simulink model "CC_CV_IR"  (R2019b)
settings: Solver=ode23s  StartTime=0.0  StopTime=96  FixedStep=50e-6  RelTol=1e-6
libraries: powerlib x14, simulink x6
settings Model: Creator=Soto Porras  LastModifiedBy=maxim
settings DataIOCC: ReturnWorkspaceOutputs=off
settings DebuggingCC: ArithmeticOperatorsInVariantConditions=warning
settings SFSimCC: CustomCodeUndefinedFunction=UseInterfaceOnly

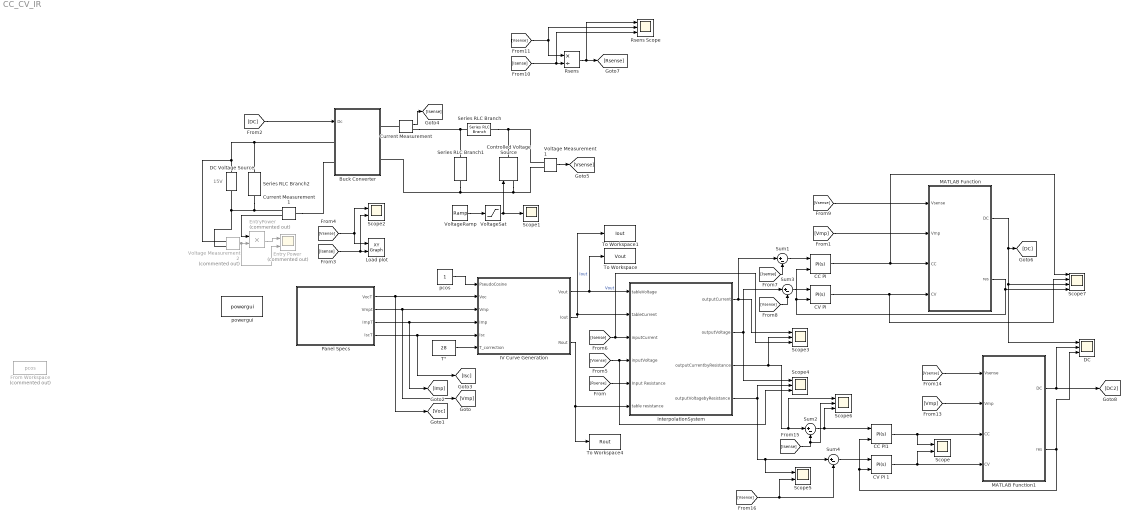
== system CC_CV_IR ==
  note: 15V
  Buck Converter : Subsystem
  CC PI : simulink/Continuous/PID Controller  Controller=PI  Form=Parallel  TimeDomain=Continuous-time  SampleTime=0.00005  IntegratorMethod=Trapezoidal  FilterMethod=Forward Euler  ControllerParametersSource=internal  P=10  I=0.01  D=0  UseFilter=on  N=100  TunerSelectOption=Frequency Response Based  InitialConditionSource=internal  InitialConditionForIntegrator=0  InitialConditionForFilter=0  DifferentiatorICPrevScaledInput=0  ExternalReset=either  TrackingMode=off  Kt=1  LimitOutput=off  UpperSaturationLimit=0.9  LowerSaturationLimit=0.1  LinearizeAsGain=on  AntiWindupMode=none  Kb=1  POutMin=[]  POutMax=[]  IOutMin=[]  IOutMax=[]  DOutMin=[]  DOutMax=[]  NOutMin=[]  NOutMax=[]  SumOutMin=[]  SumOutMax=[]  SaturationOutMin=[]  SaturationOutMax=[]  PParamMin=[]  PParamMax=[]  IParamMin=[]  IParamMax=[]  DParamMin=[]  DParamMax=[]  NParamMin=[]  NParamMax=[]  KbParamMin=[]  KbParamMax=[]  KtParamMin=[]  KtParamMax=[]  KbOutMin=[]  KbOutMax=[]  KtOutMin=[]  KtOutMax=[]  IntegratorOutMin=[]  IntegratorOutMax=[]  FilterOutMin=[]  FilterOutMax=[]  SumI1OutMin=[]  SumI1OutMax=[]  SumI2OutMin=[]  SumI2OutMax=[]  SumI3OutMin=[]  SumI3OutMax=[]  SumI4OutMin=[]  SumI4OutMax=[]  SumDOutMin=[]  SumDOutMax=[]  DifferentiatorOutMin=[]  DifferentiatorOutMax=[]  FilterDiffOutCoefMin=[]  FilterDiffOutCoefMax=[]  ReciprocalOutMin=[]  ReciprocalOutMax=[]  SumDenOutMin=[]  SumDenOutMax=[]  SumNumOutMin=[]  SumNumOutMax=[]  DivideOutMin=[]  DivideOutMax=[]  IntegratorContinuousStateAttributes=''  IntegratorStateMustResolveToSignalObject=off  IntegratorRTWStateStorageClass=Auto  FilterContinuousStateAttributes=''  FilterStateMustResolveToSignalObject=off  FilterRTWStateStorageClass=Auto  ParallelPVariant=InternalParameters  IdealPVariant=Disabled  IVariant=InternalParameters  DVariant=Disabled  IntegratorVariant=Continuous  SatVariant=Disabled  AWVariant=Passthrough  PCopyVariant=Disabled  TRVariant=Disabled  FdbkBlocksVariant=Forward  IdealPFdbkVariant=Disabled  SatFdbkVariant=Disabled  DerivativeFilterVariant=Disabled  NVariant=Disabled  NCopyVariant=Disabled_SignalSpec  FilterICVariant=Disabled  IntegratorICVariant=InternalICs  ExternalResetVariant=ExternalReset  TRSumVariant=Passthrough  SumFdbkVariant=Disabled  SumVariant=Sum_PI
  CC PI1 : simulink/Continuous/PID Controller  Controller=PI  Form=Parallel  TimeDomain=Continuous-time  SampleTime=0.00005  IntegratorMethod=Trapezoidal  FilterMethod=Forward Euler  ControllerParametersSource=internal  P=5  I=0.0001  D=0  UseFilter=on  N=100  TunerSelectOption=Frequency Response Based  InitialConditionSource=internal  InitialConditionForIntegrator=0  InitialConditionForFilter=0  DifferentiatorICPrevScaledInput=0  ExternalReset=either  TrackingMode=off  Kt=1  LimitOutput=off  UpperSaturationLimit=0.9  LowerSaturationLimit=0.1  LinearizeAsGain=on  AntiWindupMode=none  Kb=1  POutMin=[]  POutMax=[]  IOutMin=[]  IOutMax=[]  DOutMin=[]  DOutMax=[]  NOutMin=[]  NOutMax=[]  SumOutMin=[]  SumOutMax=[]  SaturationOutMin=[]  SaturationOutMax=[]  PParamMin=[]  PParamMax=[]  IParamMin=[]  IParamMax=[]  DParamMin=[]  DParamMax=[]  NParamMin=[]  NParamMax=[]  KbParamMin=[]  KbParamMax=[]  KtParamMin=[]  KtParamMax=[]  KbOutMin=[]  KbOutMax=[]  KtOutMin=[]  KtOutMax=[]  IntegratorOutMin=[]  IntegratorOutMax=[]  FilterOutMin=[]  FilterOutMax=[]  SumI1OutMin=[]  SumI1OutMax=[]  SumI2OutMin=[]  SumI2OutMax=[]  SumI3OutMin=[]  SumI3OutMax=[]  SumI4OutMin=[]  SumI4OutMax=[]  SumDOutMin=[]  SumDOutMax=[]  DifferentiatorOutMin=[]  DifferentiatorOutMax=[]  FilterDiffOutCoefMin=[]  FilterDiffOutCoefMax=[]  ReciprocalOutMin=[]  ReciprocalOutMax=[]  SumDenOutMin=[]  SumDenOutMax=[]  SumNumOutMin=[]  SumNumOutMax=[]  DivideOutMin=[]  DivideOutMax=[]  IntegratorContinuousStateAttributes=''  IntegratorStateMustResolveToSignalObject=off  IntegratorRTWStateStorageClass=Auto  FilterContinuousStateAttributes=''  FilterStateMustResolveToSignalObject=off  FilterRTWStateStorageClass=Auto  ParallelPVariant=InternalParameters  IdealPVariant=Disabled  IVariant=InternalParameters  DVariant=Disabled  IntegratorVariant=Continuous  SatVariant=Disabled  AWVariant=Passthrough  PCopyVariant=Disabled  TRVariant=Disabled  FdbkBlocksVariant=Forward  IdealPFdbkVariant=Disabled  SatFdbkVariant=Disabled  DerivativeFilterVariant=Disabled  NVariant=Disabled  NCopyVariant=Disabled_SignalSpec  FilterICVariant=Disabled  IntegratorICVariant=InternalICs  ExternalResetVariant=ExternalReset  TRSumVariant=Passthrough  SumFdbkVariant=Disabled  SumVariant=Sum_PI
  "CV PI " : simulink/Continuous/PID Controller  Controller=PI  Form=Parallel  TimeDomain=Continuous-time  SampleTime=0.00005  IntegratorMethod=Trapezoidal  FilterMethod=Forward Euler  ControllerParametersSource=internal  P=10  I=0.1  D=0.01  UseFilter=on  N=100  TunerSelectOption=Transfer Function Based (PID Tuner App)  InitialConditionSource=internal  InitialConditionForIntegrator=0  InitialConditionForFilter=0  DifferentiatorICPrevScaledInput=0  ExternalReset=either  TrackingMode=off  Kt=1  LimitOutput=off  UpperSaturationLimit=0.9  LowerSaturationLimit=0.1  LinearizeAsGain=on  AntiWindupMode=none  Kb=1  POutMin=[]  POutMax=[]  IOutMin=[]  IOutMax=[]  DOutMin=[]  DOutMax=[]  NOutMin=[]  NOutMax=[]  SumOutMin=[]  SumOutMax=[]  SaturationOutMin=[]  SaturationOutMax=[]  PParamMin=[]  PParamMax=[]  IParamMin=[]  IParamMax=[]  DParamMin=[]  DParamMax=[]  NParamMin=[]  NParamMax=[]  KbParamMin=[]  KbParamMax=[]  KtParamMin=[]  KtParamMax=[]  KbOutMin=[]  KbOutMax=[]  KtOutMin=[]  KtOutMax=[]  IntegratorOutMin=[]  IntegratorOutMax=[]  FilterOutMin=[]  FilterOutMax=[]  SumI1OutMin=[]  SumI1OutMax=[]  SumI2OutMin=[]  SumI2OutMax=[]  SumI3OutMin=[]  SumI3OutMax=[]  SumI4OutMin=[]  SumI4OutMax=[]  SumDOutMin=[]  SumDOutMax=[]  DifferentiatorOutMin=[]  DifferentiatorOutMax=[]  FilterDiffOutCoefMin=[]  FilterDiffOutCoefMax=[]  ReciprocalOutMin=[]  ReciprocalOutMax=[]  SumDenOutMin=[]  SumDenOutMax=[]  SumNumOutMin=[]  SumNumOutMax=[]  DivideOutMin=[]  DivideOutMax=[]  IntegratorContinuousStateAttributes=''  IntegratorStateMustResolveToSignalObject=off  IntegratorRTWStateStorageClass=Auto  FilterContinuousStateAttributes=''  FilterStateMustResolveToSignalObject=off  FilterRTWStateStorageClass=Auto  ParallelPVariant=InternalParameters  IdealPVariant=Disabled  IVariant=InternalParameters  DVariant=Disabled  IntegratorVariant=Continuous  SatVariant=Disabled  AWVariant=Passthrough  PCopyVariant=Disabled  TRVariant=Disabled  FdbkBlocksVariant=Forward  IdealPFdbkVariant=Disabled  SatFdbkVariant=Disabled  DerivativeFilterVariant=Disabled  NVariant=Disabled  NCopyVariant=Disabled_SignalSpec  FilterICVariant=Disabled  IntegratorICVariant=InternalICs  ExternalResetVariant=ExternalReset  TRSumVariant=Passthrough  SumFdbkVariant=Disabled  SumVariant=Sum_PI
  CV PI 1 : simulink/Continuous/PID Controller  Controller=PI  Form=Parallel  TimeDomain=Continuous-time  SampleTime=0.00005  IntegratorMethod=Trapezoidal  FilterMethod=Forward Euler  ControllerParametersSource=internal  P=10  I=0.0001  D=0.01  UseFilter=on  N=100  TunerSelectOption=Transfer Function Based (PID Tuner App)  InitialConditionSource=internal  InitialConditionForIntegrator=0  InitialConditionForFilter=0  DifferentiatorICPrevScaledInput=0  ExternalReset=either  TrackingMode=off  Kt=1  LimitOutput=off  UpperSaturationLimit=0.9  LowerSaturationLimit=0.1  LinearizeAsGain=on  AntiWindupMode=none  Kb=1  POutMin=[]  POutMax=[]  IOutMin=[]  IOutMax=[]  DOutMin=[]  DOutMax=[]  NOutMin=[]  NOutMax=[]  SumOutMin=[]  SumOutMax=[]  SaturationOutMin=[]  SaturationOutMax=[]  PParamMin=[]  PParamMax=[]  IParamMin=[]  IParamMax=[]  DParamMin=[]  DParamMax=[]  NParamMin=[]  NParamMax=[]  KbParamMin=[]  KbParamMax=[]  KtParamMin=[]  KtParamMax=[]  KbOutMin=[]  KbOutMax=[]  KtOutMin=[]  KtOutMax=[]  IntegratorOutMin=[]  IntegratorOutMax=[]  FilterOutMin=[]  FilterOutMax=[]  SumI1OutMin=[]  SumI1OutMax=[]  SumI2OutMin=[]  SumI2OutMax=[]  SumI3OutMin=[]  SumI3OutMax=[]  SumI4OutMin=[]  SumI4OutMax=[]  SumDOutMin=[]  SumDOutMax=[]  DifferentiatorOutMin=[]  DifferentiatorOutMax=[]  FilterDiffOutCoefMin=[]  FilterDiffOutCoefMax=[]  ReciprocalOutMin=[]  ReciprocalOutMax=[]  SumDenOutMin=[]  SumDenOutMax=[]  SumNumOutMin=[]  SumNumOutMax=[]  DivideOutMin=[]  DivideOutMax=[]  IntegratorContinuousStateAttributes=''  IntegratorStateMustResolveToSignalObject=off  IntegratorRTWStateStorageClass=Auto  FilterContinuousStateAttributes=''  FilterStateMustResolveToSignalObject=off  FilterRTWStateStorageClass=Auto  ParallelPVariant=InternalParameters  IdealPVariant=Disabled  IVariant=InternalParameters  DVariant=Disabled  IntegratorVariant=Continuous  SatVariant=Disabled  AWVariant=Passthrough  PCopyVariant=Disabled  TRVariant=Disabled  FdbkBlocksVariant=Forward  IdealPFdbkVariant=Disabled  SatFdbkVariant=Disabled  DerivativeFilterVariant=Disabled  NVariant=Disabled  NCopyVariant=Disabled_SignalSpec  FilterICVariant=Disabled  IntegratorICVariant=InternalICs  ExternalResetVariant=ExternalReset  TRSumVariant=Passthrough  SumFdbkVariant=Disabled  SumVariant=Sum_PI
  Controlled Voltage Source : powerlib/Electrical Sources/Controlled Voltage Source  Initialize=on  Source_Type=DC  Amplitude=0.1  Phase=0  Frequency=0  Measurements=None
      settings: SourceProductName=Simscape Electrical
  Current Measurement : powerlib/Measurements/Current Measurement  PhasorSimulation=off  OutputType=Complex  PSBequivalent=0
      settings: SourceProductName=Simscape Electrical
  Current Measurement1 : powerlib/Measurements/Current Measurement  PhasorSimulation=off  OutputType=Complex  PSBequivalent=0
      settings: SourceProductName=Simscape Electrical
  "DC " : Scope  NumInputPorts=3
  DC Voltage Source : powerlib/Electrical Sources/DC Voltage Source  Amplitude=15  Measurements=None
      settings: SourceProductName=Simscape Electrical
  "Entry Power " : Scope  Commented=on  NumInputPorts=2
  EntryPower : Product  Commented=on
  From Workspace : FromWorkspace  Commented=on  VariableName=pcos  SampleTime=0
  IV Curve Generation : Subsystem  mask(Panel I-V Curve Calculation){ValueVocComp=0.0062, ValueVmpComp=0.0067}
      mask prompts: ValueVocComp "Voc Temperature Correction (V)"; ValueVmpComp "Vmp Temperature Correction (V)"
      mask help:
      | This module calculates the panel IV curve using the next panel parameters:
      | 1. Voc
      | 2. Vmp
      | 3. Imp
      | 4. Isc
      |
      | It applies:
      | 1. Correction to current parameters (Isc and Imp) using a pseudo cosine that varies depending on the angle of the perpendicular CubeSat face and the sun's incident radiation.
      | 2. Correction to voltage parameters (Voc and Vmp) using the panel datasheet voltage losses, given in V by the user.
      mask TypeOptions ValueVocComp: Voc_comp/Value
      mask TypeOptions ValueVmpComp: Vmp_comp/Value
      mask Display: image('IV_curve.png');
  InterpolationSystem : Subsystem
  Load plot : simulink/Sinks/XY Graph  xmin=0  xmax=6  ymin=0  ymax=2  st=-1
  MATLAB Function : MATLAB Function  TreatAsAtomicUnit=on
  MATLAB Function1 : MATLAB Function  TreatAsAtomicUnit=on
  Panel Specs : Subsystem  mask(Solar Panel Specifications){Voc=2.690, Vmp=2.409, Imp=0.5029, Isc=0.5196, SerialGain=2, ParallelGain=3}
      mask prompts: SerialGain "Serial"; ParallelGain "Parallel"
      mask help: Inputs solar panel electrical specifications, temperature and array distribution.
      mask TypeOptions Voc: Voc/Value
      mask TypeOptions Vmp: Vmp/Value
      mask TypeOptions Imp: Imp/Value
      mask TypeOptions Isc: Isc/Value
      mask TypeOptions SerialGain: Gain/Gain | Gain1/Gain
      mask TypeOptions ParallelGain: Gain2/Gain | Gain3/Gain
      mask DialogControl Container3 Prompt: Panel Array
      mask Display: image('solar_panel.png');
  Rsens : Product  Inputs=*/
  Rsens Scope : Scope  NumInputPorts=3
  Scope : Scope  NumInputPorts=2
  Scope1 : Scope
  Scope2 : Scope  NumInputPorts=2
  Scope3 : Scope  NumInputPorts=3
  Scope4 : Scope  NumInputPorts=3
  Scope5 : Scope  NumInputPorts=2
  Scope6 : Scope  NumInputPorts=3
  Scope7 : Scope  NumInputPorts=4
  Series RLC Branch : powerlib/Elements/Series RLC Branch  LConnTagsString=__new0  RConnTagsString=__new0  BranchType=R  Resistance=1e-3  Inductance=1e-3  SetiL0=off  InitialCurrent=0  Capacitance=1e-6  Setx0=off  InitialVoltage=0  Measurements=None
      settings: SourceProductName=Simscape Electrical
  Series RLC Branch1 : powerlib/Elements/Series RLC Branch  LConnTagsString=__new0  RConnTagsString=__new0  BranchType=RC  Resistance=1e-2  Inductance=1e-3  SetiL0=off  InitialCurrent=0  Capacitance=100e-6  Setx0=off  InitialVoltage=0  Measurements=None
      settings: SourceProductName=Simscape Electrical
  Series RLC Branch2 : powerlib/Elements/Series RLC Branch  LConnTagsString=__new0  RConnTagsString=__new0  BranchType=RC  Resistance=1e-3  Inductance=1e-3  SetiL0=off  InitialCurrent=0  Capacitance=100e-6  Setx0=off  InitialVoltage=0  Measurements=None
      settings: SourceProductName=Simscape Electrical
  Sum{1..4} (4 alike) : Sum  Inputs=|+-
  To Workspace : ToWorkspace  VariableName=Vout  SaveFormat=Structure With Time  SampleTime=-1
  To Workspace1 : ToWorkspace  VariableName=Iout  SaveFormat=Structure With Time  SampleTime=-1
  To Workspace4 : ToWorkspace  VariableName=Rout  SaveFormat=Structure With Time  SampleTime=-1
  T° : Constant  Value=28
  Voltage Measurement1 : powerlib/Measurements/Voltage Measurement  PhasorSimulation=off  OutputType=Complex  PSBequivalent=0
      settings: SourceProductName=Simscape Electrical
  Voltage Measurement2 : powerlib/Measurements/Voltage Measurement  Commented=on  PhasorSimulation=off  OutputType=Complex  PSBequivalent=0
      settings: SourceProductName=Simscape Electrical
  VoltageRamp : simulink/Sources/Ramp  slope=0.0538  start=0  InitialOutput=0
  VoltageSat : Saturate  UpperLimit=5.38  LowerLimit=0
  pcos : Constant
  powergui : powerlib/powergui  Priority=1  SimulationMode=Continuous  SampleTime=50e-6  frequency=60  Iterations=50  frequencyindice=0  Pbase=100e6  ErrMax=1e-4  UnitsV=kV  UnitsW=MW  buscounter=0  FunctionMessages=off  echomessages=off  EnableUseOfTLC=off  CurrentSourceSwitches=off  DisableSnubberDevices=off  DisableRonSwitches=off  DisableVfSwitches=off  DisplayEquations=off  AutomaticDiscreteSolvers=off  SolverType=Tustin/Backward Euler (TBE)  Interpol=off  ExternalGateDelay=off  methode=off  Ts=100  x0status=blocks  SPID=on  SwTol=0  HookPort=off  NonlinearTolerance=0  nMaxIteration=15  ContinueOnMaxIteration=off  RestoreLinks=warning  ResistiveCurrentMeasurement=off  Frange=[0:2:500]  Ylog=off  Xlog=on  ShowGrid=off  save=off  variable=ZData  structure=0  ZoomFFT=off  StartTime=0.0  cycles=1  DisplayStyle=1  fundamental=60  FreqAxis=off  MaxFrequency=1000  frequencyindicesteady=1  RmsSteady=1  display=off
      settings: SourceProductName=Simscape Electrical
  wires:
  Panel Specs/1(VocT) -> IV Curve Generation/2(Voc), [Voc]
  Panel Specs/2(Vmpt) -> IV Curve Generation/3(Vmp), [Vmp]
  Panel Specs/3(ImpT) -> IV Curve Generation/4(Imp), [Imp]
  Panel Specs/4(IscT) -> [Isc], IV Curve Generation/5(Isc)
  IV Curve Generation/1(Vout) -> To Workspace/1, InterpolationSystem/1(tableVoltage)  "Vout"
  IV Curve Generation/2(Iout) -> To Workspace1/1, InterpolationSystem/2(tableCurrent)  "Iout"
  T°/1 -> IV Curve Generation/6(T_correction)
  Sum1/1 -> CC PI/1
  VoltageSat/1 -> Scope1/1, Controlled Voltage Source/1
  Voltage Measurement1/1 -> [Vsense]
  InterpolationSystem/1(outputCurrent) -> Sum1/1, Scope3/1
  CC PI/1 -> Scope7/1, MATLAB Function/3(CC)
  "CV PI "/1 -> Scope7/2, MATLAB Function/4(CV)
  Sum3/1 -> "CV PI "/1
  [Isense] -> Scope2/2, Load plot/2
  [Vsense] -> Scope2/1, Load plot/1
  [Vsense] -> Scope4/3, InterpolationSystem/4(inputVoltage)
  [Isense] -> Scope3/3, InterpolationSystem/3(inputCurrent)
  [Isense] -> Sum1/2
  [Vsense] -> Sum3/2
  [Vsense] -> MATLAB Function/1(Vsense)
  [Vmp] -> MATLAB Function/2(Vmp)
  pcos/1 -> IV Curve Generation/1(PseudoCosine)
  VoltageRamp/1 -> VoltageSat/1
  Current Measurement/1 -> [Isense]
  MATLAB Function/1(DC) -> "DC "/1, Scope7/3, [DC]
  [DC] -> Buck Converter/1(Dc)
  IV Curve Generation/3("Rout ") -> To Workspace4/1, InterpolationSystem/6(table resistance)
  Rsens/1 -> Rsens Scope/1, [Rsense]
  [Isense] -> Rsens Scope/3, Rsens/2
  [Vsense] -> Rsens/1, Rsens Scope/2
  [Rsense] -> InterpolationSystem/5(Input Resistance)
  InterpolationSystem/3("outputCurrentbyResistance ") -> Scope6/1, Sum2/1, Scope3/2
  InterpolationSystem/2(outputVoltage) -> Scope4/1, Sum3/1
  Current Measurement1/1 -> EntryPower/1
  Voltage Measurement2/1 -> "Entry Power "/2, EntryPower/2
  EntryPower/1 -> "Entry Power "/1
  MATLAB Function/2(res) -> Scope7/4, CC PI/2, "CV PI "/2
  InterpolationSystem/4(outputVoltagebyResistance) -> Scope5/1, Sum4/1, Scope4/2
  MATLAB Function1/1(DC) -> "DC "/2, [DC2]
  [Vsense] -> MATLAB Function1/1(Vsense)
  [Vmp] -> MATLAB Function1/2(Vmp)
  CV PI 1/1 -> Scope/2, MATLAB Function1/4(CV)
  CC PI1/1 -> Scope/1, MATLAB Function1/3(CC)
  MATLAB Function1/2(res) -> CC PI1/2, CV PI 1/2, "DC "/3
  [Isense] -> Scope6/2, Sum2/2
  Sum2/1 -> CC PI1/1, Scope6/3
  [Vsense] -> Scope5/2, Sum4/2
  Sum4/1 -> CV PI 1/1
  connections:
  DC Voltage Source/RConn1 -- Series RLC Branch2/LConn1 -- Buck Converter/LConn1 -- Voltage Measurement2/LConn1
  Series RLC Branch2/RConn1 -- Voltage Measurement2/LConn2 -- DC Voltage Source/LConn1 -- Current Measurement1/RConn1
  Voltage Measurement1/LConn2 -- Controlled Voltage Source/LConn1 -- Buck Converter/RConn2 -- Series RLC Branch1/RConn1
  Series RLC Branch/LConn1 -- Voltage Measurement1/LConn1 -- Controlled Voltage Source/RConn1
  Current Measurement/LConn1 -- Buck Converter/RConn1
  Current Measurement/RConn1 -- Series RLC Branch1/LConn1 -- Series RLC Branch/RConn1
  Current Measurement1/LConn1 -- Buck Converter/LConn2

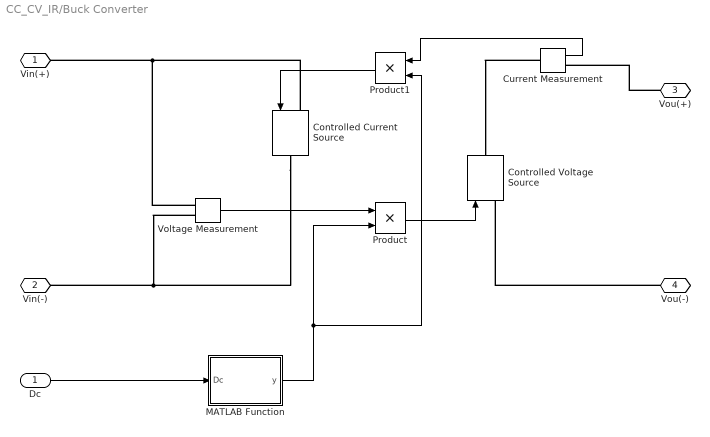
== system CC_CV_IR/Buck Converter ==
  Dc : Inport
  Controlled Current Source : powerlib/Electrical Sources/Controlled Current Source  Initialize=off  Source_Type=DC  Amplitude=0  Phase=0  Frequency=0  Measurements=None
      settings: SourceProductName=Simscape Electrical
  Controlled Voltage Source : powerlib/Electrical Sources/Controlled Voltage Source  Initialize=off  Source_Type=DC  Amplitude=0  Phase=0  Frequency=0  Measurements=None
      settings: SourceProductName=Simscape Electrical
  Current Measurement : powerlib/Measurements/Current Measurement  PhasorSimulation=off  OutputType=Complex  PSBequivalent=0
      settings: SourceProductName=Simscape Electrical
  MATLAB Function : MATLAB Function  TreatAsAtomicUnit=on
  Product : Product
  Product1 : Product
  Voltage Measurement : powerlib/Measurements/Voltage Measurement  PhasorSimulation=off  OutputType=Complex  PSBequivalent=0
      settings: SourceProductName=Simscape Electrical
  Vin(+) : PMIOPort  Side=Left
  Vin(-) : PMIOPort  Port=2  Side=Left
  Vou(+) : PMIOPort  Port=3  Side=Right
  Vou(-) : PMIOPort  Port=4  Side=Right
  wires:
  Current Measurement/1 -> Product1/1
  MATLAB Function/1(y) -> Product1/2, Product/2
  Voltage Measurement/1 -> Product/1
  Dc/1 -> MATLAB Function/1(Dc)
  Product/1 -> Controlled Voltage Source/1
  Product1/1 -> Controlled Current Source/1
  connections:
  Controlled Current Source/RConn1 -- Voltage Measurement/LConn2 -- Vin(-)/RConn1
  Vou(-)/RConn1 -- Controlled Voltage Source/LConn1
  Current Measurement/LConn1 -- Controlled Voltage Source/RConn1
  Controlled Current Source/LConn1 -- Voltage Measurement/LConn1 -- Vin(+)/RConn1
  Vou(+)/RConn1 -- Current Measurement/RConn1

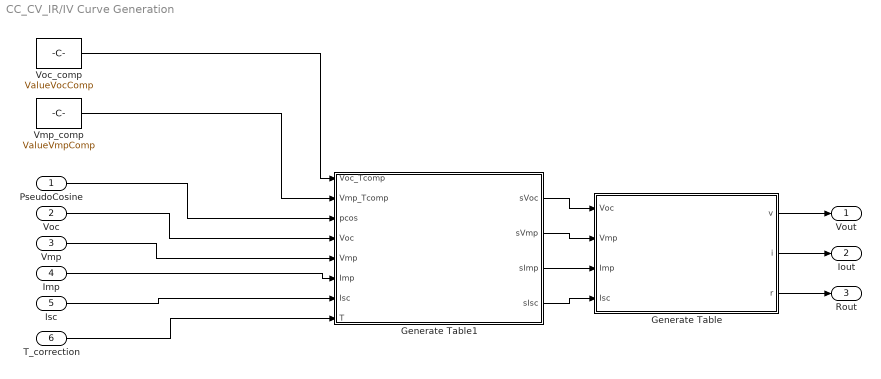
== system CC_CV_IR/IV Curve Generation ==
  PseudoCosine : Inport
  Voc : Inport  Port=2
  Vmp : Inport  Port=3
  Imp : Inport  Port=4
  Isc : Inport  Port=5
  T_correction : Inport  Port=6
  Generate Table : MATLAB Function  TreatAsAtomicUnit=on
  Generate Table1 : MATLAB Function  TreatAsAtomicUnit=on
  Vmp_comp : Constant  Value=ValueVmpComp
  Voc_comp : Constant  Value=ValueVocComp
  Vout : Outport  VectorParamsAs1DForOutWhenUnconnected=off
  Iout : Outport  Port=2  VectorParamsAs1DForOutWhenUnconnected=off
  "Rout " : Outport  Port=3  VectorParamsAs1DForOutWhenUnconnected=off
  wires:
  Isc/1 -> Generate Table1/7(Isc)
  Generate Table1/4(sIsc) -> Generate Table/4(Isc)
  Voc_comp/1 -> Generate Table1/1(Voc_Tcomp)
  Generate Table/1(v) -> Vout/1
  T_correction/1 -> Generate Table1/8(T)
  Generate Table1/2(sVmp) -> Generate Table/2(Vmp)
  Voc/1 -> Generate Table1/4(Voc)
  Generate Table1/3(sImp) -> Generate Table/3(Imp)
  Imp/1 -> Generate Table1/6(Imp)
  Generate Table1/1(sVoc) -> Generate Table/1(Voc)
  Vmp/1 -> Generate Table1/5(Vmp)
  Generate Table/2(i) -> Iout/1
  Vmp_comp/1 -> Generate Table1/2(Vmp_Tcomp)
  PseudoCosine/1 -> Generate Table1/3(pcos)
  Generate Table/3(r) -> "Rout "/1

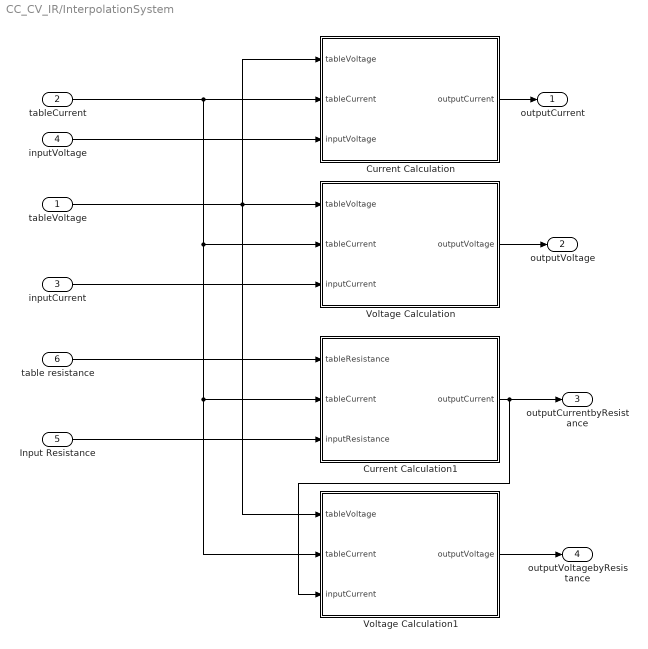
== system CC_CV_IR/InterpolationSystem ==
  tableVoltage : Inport
  tableCurrent : Inport  Port=2
  inputCurrent : Inport  Port=3
  inputVoltage : Inport  Port=4
  Input Resistance : Inport  Port=5
  table resistance : Inport  Port=6
  Current Calculation : MATLAB Function  TreatAsAtomicUnit=on
  Current Calculation1 : MATLAB Function  TreatAsAtomicUnit=on
  Voltage Calculation : MATLAB Function  TreatAsAtomicUnit=on
  Voltage Calculation1 : MATLAB Function  TreatAsAtomicUnit=on
  outputCurrent : Outport  VectorParamsAs1DForOutWhenUnconnected=off
  outputVoltage : Outport  Port=2  VectorParamsAs1DForOutWhenUnconnected=off
  "outputCurrentbyResistance " : Outport  Port=3  VectorParamsAs1DForOutWhenUnconnected=off
  outputVoltagebyResistance : Outport  Port=4  VectorParamsAs1DForOutWhenUnconnected=off
  wires:
  Voltage Calculation/1(outputVoltage) -> outputVoltage/1
  tableVoltage/1 -> Voltage Calculation1/1(tableVoltage), Voltage Calculation/1(tableVoltage), Current Calculation/1(tableVoltage)
  Current Calculation/1(outputCurrent) -> outputCurrent/1
  tableCurrent/1 -> Voltage Calculation1/2(tableCurrent), Current Calculation1/2(tableCurrent), Voltage Calculation/2(tableCurrent), Current Calculation/2(tableCurrent)
  inputCurrent/1 -> Voltage Calculation/3(inputCurrent)
  inputVoltage/1 -> Current Calculation/3(inputVoltage)
  Input Resistance/1 -> Current Calculation1/3(inputResistance)
  table resistance/1 -> Current Calculation1/1(tableResistance)
  Current Calculation1/1(outputCurrent) -> Voltage Calculation1/3(inputCurrent), "outputCurrentbyResistance "/1
  Voltage Calculation1/1(outputVoltage) -> outputVoltagebyResistance/1

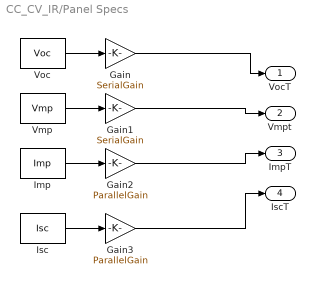
== system CC_CV_IR/Panel Specs ==
  Gain : Gain  Gain=SerialGain
  Gain1 : Gain  Gain=SerialGain
  Gain2 : Gain  Gain=ParallelGain
  Gain3 : Gain  Gain=ParallelGain
  Imp : Constant  Value=Imp
  Isc : Constant  Value=Isc
  Vmp : Constant  Value=Vmp
  Voc : Constant  Value=Voc
  VocT : Outport  VectorParamsAs1DForOutWhenUnconnected=off
  Vmpt : Outport  Port=2  VectorParamsAs1DForOutWhenUnconnected=off
  ImpT : Outport  Port=3  VectorParamsAs1DForOutWhenUnconnected=off
  IscT : Outport  Port=4  VectorParamsAs1DForOutWhenUnconnected=off
  wires:
  Isc/1 -> Gain3/1
  Vmp/1 -> Gain1/1
  Gain/1 -> VocT/1
  Imp/1 -> Gain2/1
  Gain2/1 -> ImpT/1
  Gain3/1 -> IscT/1
  Voc/1 -> Gain/1
  Gain1/1 -> Vmpt/1

== matlab function CC_CV_IR/Buck Converter/MATLAB Function ==
  data: Dc input; y output
function y = M(Dc)
y = Dc;

== matlab function CC_CV_IR/InterpolationSystem/Voltage Calculation ==
  data: outputVoltage output; tableVoltage input; tableCurrent input; inputCurrent input
function outputVoltage  = CurrentInverseInterpolation(tableVoltage, tableCurrent, inputCurrent)
    
    % Apply inverse interpolation on ampere ramp values
    n = 1024;
    v = 0;
    %i = 1023;
    for j = 1 : n - 1
        i = 1024 - j;
        if(inputCurrent < tableCurrent(i))
           v = tableVoltage(i) + (tableVoltage(i+1)-tableVoltage(i))*((inputCurrent - tableCurrent(i))/(tableCurrent(i+1) - tableCurrent(i)));
           break;
        end
    end
    outputVoltage = v;
    
end

== matlab function CC_CV_IR/IV Curve Generation/Generate Table ==
  data: Voc input; Vmp input; Imp input; Isc input; v output; i output; r output
function [v,i,r] = generate_table(Voc, Vmp, Imp, Isc)
Rs = ( Voc - Vmp ) / Imp;
a = ( Vmp * ( 1 + ( Rs*Isc ) / Voc ) + Rs*( Imp - Isc ) ) / Voc;
N = log( 2 - 2^a) / log ( Imp / Isc );
i=zeros(1024,1);
v=zeros(1024,1);
r=zeros(1024,1);
for x = 1:1024
    I = (x * Isc) / 1023.0;
    V = Voc * log( 2 - ( ( I / Isc ) ^ N ) );
    V = V / log( 2 );
    V = V - Rs * ( I - Isc );
    V = V / ( 1 + ( ( Rs * Isc) / Voc) );
    P = V * I;
    v(x) = V;
    i(x) = I;
    if i(x) == 0
        r(i) = 1000;
    else
        r(x) = v(x)/i(x);
    end 
end
v = flip(v);
i = flip(i);
r = flip(r);

== matlab function CC_CV_IR/InterpolationSystem/Current Calculation ==
  data: outputCurrent output; tableVoltage input; tableCurrent input; inputVoltage input
function outputCurrent  = VoltageInterpolation(tableVoltage, tableCurrent, inputVoltage)
    
    % Apply interpolation on voltage ramp values
    n = 1023;
    c = 0;
    for j = 1 : n + 1
        i = j;
        if(inputVoltage < tableVoltage(i))
           c = tableCurrent(i) + ...
               (tableCurrent(i-1)-tableCurrent(i))*...
               ((inputVoltage - tableVoltage(i))/(tableVoltage(i-1) - tableVoltage(i)));
           break;
        end
    end
    outputCurrent = c;
    
end

== matlab function CC_CV_IR/MATLAB Function ==
  data: Vsense input; Vmp input; CC input; DC output; CV input; res output
function [DC, res]= CC_CV(Vsense,Vmp,CC,CV)

    if Vsense >= Vmp
        DC = CV;
        res = 1;
    else 
        DC = CC;
        res = 0;
end

== matlab function CC_CV_IR/IV Curve Generation/Generate Table1 ==
  data: Voc_Tcomp input; Vmp_Tcomp input; pcos input; Voc input; Vmp input; Imp input; Isc input; sVoc output; sVmp output; sImp output; sIsc output; T input
function [sVoc, sVmp, sImp, sIsc] = scalevars(Voc_Tcomp, Vmp_Tcomp, pcos, Voc, Vmp, Imp, Isc, T)
sVoc = Voc-(T*Voc_Tcomp);
sVmp = Vmp-(T*Vmp_Tcomp);
sImp = pcos * Imp;
sIsc = pcos * Isc;

== matlab function CC_CV_IR/InterpolationSystem/Current Calculation1 ==
  data: tableResistance input; outputCurrent output; tableCurrent input; inputResistance input
function outputCurrent  = ResistanceInterpolation(tableResistance, tableCurrent, inputResistance)

    % Apply interpolation on voltage ramp values
    n = 1023;
    c = 0;
    for j = 2 : n + 1
        i = j;
        if(inputResistance < tableResistance(i))
           c = tableCurrent(i) + ...
               (tableCurrent(i-1)-tableCurrent(i))*...
               ((inputResistance - tableResistance(i))/(tableResistance(i-1) - tableResistance(i)));
           break;
        end
    end
    outputCurrent = c;
    
end

== matlab function CC_CV_IR/InterpolationSystem/Voltage Calculation1 ==
  data: outputVoltage output; tableVoltage input; tableCurrent input; inputCurrent input
function outputVoltage  = CurrentInverseInterpolation(tableVoltage, tableCurrent, inputCurrent)
    
    % Apply inverse interpolation on ampere ramp values
    n = 1024;
    v = 0;
    %i = 1023;
    for j = 1 : n - 1
        i = 1024 - j;
        if(inputCurrent < tableCurrent(i))
           v = tableVoltage(i) + (tableVoltage(i+1)-tableVoltage(i))*((inputCurrent - tableCurrent(i))/(tableCurrent(i+1) - tableCurrent(i)));
           break;
        end
    end
    outputVoltage = v;
    
end

== matlab function CC_CV_IR/MATLAB Function1 ==
  data: Vsense input; Vmp input; CC input; DC output; CV input; res output
function [DC, res]= CC_CV_2(Vsense,Vmp,CC,CV)

    if Vsense >= Vmp
        DC = CV;
        res = 1;
    else 
        DC = CC;
        res = 0;
end
